simulink model "Furuta_Pendulum_Model_Revolinsky_V4"  (R2018b)
settings: Solver=ode1  StartTime=0.0  StopTime=inf  FixedStep=0.002  RelTol=1e-3  EnableMultiTasking=on
PostLoadFcn:
  | qc_set_target_type(getConfigSet(bdroot, 'QUARC Default Target Configuration'));
values from neighbouring files (symbols this model uses):
  A = zeros(4)    [Furuta_Pendulum_setup_Revolinsky.m]    (also in Furuta_Pendulum_setup_Revolinsky_edited.m; Matlab_MECA_482_SP20_Furuta_Revolinsky.m)
  a_max = T_max./(m_r.*L_r)    [Furuta_Pendulum_setup_Revolinsky.m]    (also in Furuta_Pendulum_setup_Revolinsky_edited.m; Matlab_MECA_482_SP20_Furuta_Revolinsky.m = 0)
  B = K_g * k_t * B / R_m    [Furuta_Pendulum_setup_Revolinsky.m]    (also in Furuta_Pendulum_setup_Revolinsky_edited.m; Matlab_MECA_482_SP20_Furuta_Revolinsky.m = zeros(1,4)')
  C = zeros(2,4)    [Furuta_Pendulum_setup_Revolinsky.m]    (also in Furuta_Pendulum_setup_Revolinsky_edited.m; Matlab_MECA_482_SP20_Furuta_Revolinsky.m)
  D = zeros(1,2)'    [Furuta_Pendulum_setup_Revolinsky.m]    (also in Furuta_Pendulum_setup_Revolinsky_edited.m; Matlab_MECA_482_SP20_Furuta_Revolinsky.m)
  epsilon = 12.0 * pi / 180    (= 0.209439510239)    [Furuta_Pendulum_setup_Revolinsky.m]    (also in Furuta_Pendulum_setup_Revolinsky_edited.m; Matlab_MECA_482_SP20_Furuta_Revolinsky.m)
  Er = Ep_upright_position    [Furuta_Pendulum_setup_Revolinsky.m]    (also in Furuta_Pendulum_setup_Revolinsky_edited.m; Matlab_MECA_482_SP20_Furuta_Revolinsky.m = 0)
  g = 9.81    [Furuta_Pendulum_setup_Revolinsky.m]    (also in Furuta_Pendulum_setup_Revolinsky_edited.m; Matlab_MECA_482_SP20_Furuta_Revolinsky.m)
  J_p = m_p .* L_p.^2 ./ 12    [Furuta_Pendulum_setup_Revolinsky.m]    (also in Furuta_Pendulum_setup_Revolinsky_edited.m; Matlab_MECA_482_SP20_Furuta_Revolinsky.m)
  K_g = Kgi * Kge    (= 70)    [Furuta_Pendulum_setup_Revolinsky.m]    (also in Furuta_Pendulum_setup_Revolinsky_edited.m; Matlab_MECA_482_SP20_Furuta_Revolinsky.m)
  k_m = 0.804 / 1000 * (60 / ( 2 * pi ))    (= 0.00767763445475)    [Furuta_Pendulum_setup_Revolinsky.m]    (also in Furuta_Pendulum_setup_Revolinsky_edited.m; Matlab_MECA_482_SP20_Furuta_Revolinsky.m)
  k_t = 1.088 * 0.2780139 * 0.0254    (= 0.00768296972928)    [Furuta_Pendulum_setup_Revolinsky.m]    (also in Furuta_Pendulum_setup_Revolinsky_edited.m; Matlab_MECA_482_SP20_Furuta_Revolinsky.m)
  L_p = 0.33655    [Furuta_Pendulum_setup_Revolinsky.m]    (also in Furuta_Pendulum_setup_Revolinsky_edited.m; Matlab_MECA_482_SP20_Furuta_Revolinsky.m)
  L_r = 0.2159    [Furuta_Pendulum_setup_Revolinsky.m]    (also in Furuta_Pendulum_setup_Revolinsky_edited.m; Matlab_MECA_482_SP20_Furuta_Revolinsky.m)
  m_p = 0.127    [Furuta_Pendulum_setup_Revolinsky.m]    (also in Furuta_Pendulum_setup_Revolinsky_edited.m; Matlab_MECA_482_SP20_Furuta_Revolinsky.m)
  m_r = 0.257    [Furuta_Pendulum_setup_Revolinsky.m]    (also in Furuta_Pendulum_setup_Revolinsky_edited.m; Matlab_MECA_482_SP20_Furuta_Revolinsky.m)
  n_g = 0.9    [Furuta_Pendulum_setup_Revolinsky.m]    (also in Furuta_Pendulum_setup_Revolinsky_edited.m; Matlab_MECA_482_SP20_Furuta_Revolinsky.m)
  n_m = 0.69    [Furuta_Pendulum_setup_Revolinsky.m]    (also in Furuta_Pendulum_setup_Revolinsky_edited.m; Matlab_MECA_482_SP20_Furuta_Revolinsky.m)
  R_m = 2.6    [Furuta_Pendulum_setup_Revolinsky.m]    (also in Furuta_Pendulum_setup_Revolinsky_edited.m; Matlab_MECA_482_SP20_Furuta_Revolinsky.m)
  wcf_1 = 2 * pi * 10.0    (= 62.8318530718)    [Furuta_Pendulum_setup_Revolinsky.m]    (also in Furuta_Pendulum_setup_Revolinsky_edited.m; Matlab_MECA_482_SP20_Furuta_Revolinsky.m)
  wcf_2 = 2 * pi * 10.0    (= 62.8318530718)    [Furuta_Pendulum_setup_Revolinsky.m]    (also in Furuta_Pendulum_setup_Revolinsky_edited.m; Matlab_MECA_482_SP20_Furuta_Revolinsky.m)
undefined symbols (not defined in the file or in its folder): K
libraries: simulink_extras x3, simulink x3
settings Model: ExtModeTrigDuration=10000  Creator=MLevis  LastModifiedBy=revol
settings SolverCC: PositivePriorityOrder=on
settings DataIOCC: LimitDataPoints=on  SaveFormat=Array  SignalLoggingSaveFormat=ModelDataLogs  ReturnWorkspaceOutputs=on
settings OptimizationCC: ExpressionDepthLimit=2147483647  InitFltsAndDblsToZero=on  LifeSpan=inf
settings DebuggingCC: SaveWithParameterizedLinksMsg=none  UnderspecifiedInitializationDetection=Classic  MergeDetectMultiDrivingBlocksExec=none  SolverPrmCheckMsg=warning  MultiTaskDSMMsg=warning  MultiTaskCondExecSysMsg=none  FcnCallInpInsideContextMsg=warning  StateNameClashWarn=warning  SFUnexpectedBacktrackingDiag=warning  SFNoUnconditionalDefaultTransitionDiag=warning  SFExecutionAtInitializationDiag=none
settings HardwareCC: ProdBitPerPointer=32  ProdBitPerSizeT=32  ProdBitPerPtrDiffT=32  ProdLargestAtomicFloat=None  ProdIntDivRoundTo=Undefined  ProdEndianess=Unspecified  ProdWordSize=32  ProdHWDeviceType=32-bit Generic
settings ModelReferenceCC: PropagateSignalLabelsOutOfModel=off
settings SFSimCC: SimUseLocalCustomCode=off
settings RTWCC: SystemTargetFile=quarc_win64.tlc  TemplateMakefile=quarc_default_tmf  Description=QUARC Win64 Target  RTWUseLocalCustomCode=off
settings CodeAppCC: StateflowObjectComments=on
settings STFCustomTargetCC: TargetPreCompLibLocation=C:\PROGRA~3\QUARC\lib\2018b\win64\release  GeneratePreprocessorConditionals=Disable all  CPPClassGenCompliant=on  GRTInterface=on  SystemTargetFile=quarc_win64.tlc
settings GRTTargetCC: TargetPreCompLibLocation=C:\PROGRA~3\QUARC\lib\2018b\win64\release  TargetLangStandard=C89/C90 (ANSI)  ParMdlRefBuildCompliant=off  CompOptLevelCompliant=off  ConcurrentExecutionCompliant=off  GeneratePreprocessorConditionals=Disable all  CombineOutputUpdateFcns=off  MatFileLogging=off  GRTInterface=on  UseToolchainInfoCompliant=off  ExtMode=on  ExtModeMexFile=quarc_comm
settings ConfigComp: CovMetricSettings=dw  CovHtmlReporting=on  CovSaveCumulativeToWorkspaceVar=on  CovSaveSingleToWorkspaceVar=on  CovExternalEMLEnable=off

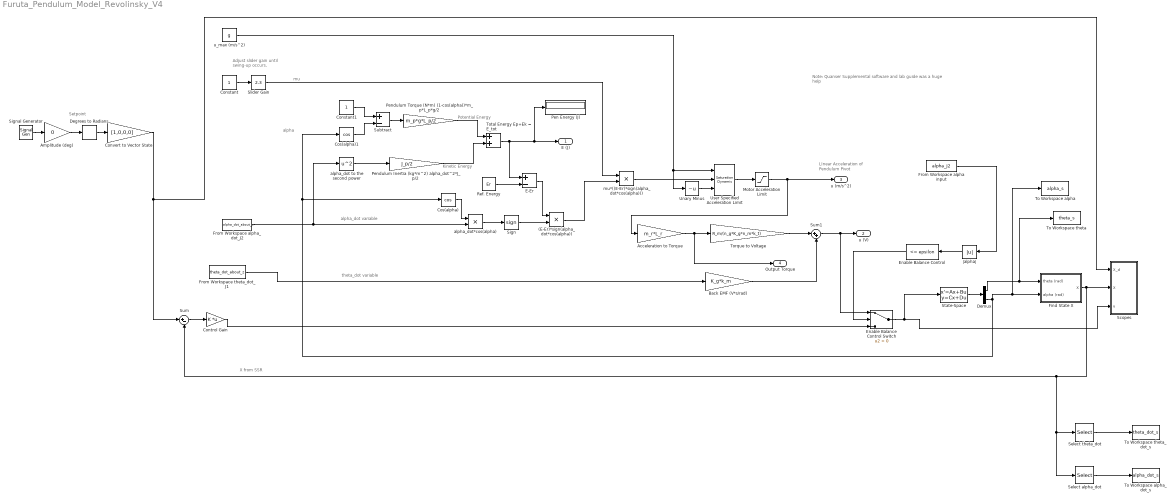
== system Furuta_Pendulum_Model_Revolinsky_V4 ==
  note: Setpoint
  note: Adjust slider gain
      | until swing-up occurs.
  note: theta_dot variable
  note: LInear Acceleration of
      | Pendulum Pivot
  note: Potential Energy
  note: Kinetic Energy
  note: alpha_dot variable
  note: X from SSR
  note: alpha
  note: mu
  note: Note: Quanser Supplemental software and lab guide was a huge help
  (E-Er)*sign(alpha_dot*cos(alpha)) : Product
  Acceleration to Torque : Gain  Gain=m_r*L_r
  Amplitude (deg) : Gain  Gain=0  SaturateOnIntegerOverflow=on  OutDataTypeStr=Inherit: Same as input  ParamDataTypeStr=Inherit: Same as input
  Back EMF (V*s/rad) : Gain  Gain=K_g*k_m
  Constant : Constant
  Constant1 : Constant
  Control Gain : Gain  Gain=K  Multiplication=Matrix(K*u)
  Convert to Vector State : Gain  Gain=[1,0,0,0]
  Cos(alpha) : Trigonometry  Operator=cos
  Cos(alpha)1 : Trigonometry  Operator=cos
  Degrees to Radians : simulink_extras/Transformations/Degrees to Radians
  Demux : Demux  Outputs=2
  E-Er : Sum  Inputs=+-
  Enable Balance Control : simulink/Logic and Bit Operations/Compare To Constant  relop=<=  const=epsilon  OutDataTypeStr=uint8  ZeroCross=off
  Enable Balance Control Switch : Switch  Criteria=u2 > Threshold
  Find State X : Subsystem
  From Workspace alpha input : FromWorkspace  VariableName=alpha_J2
  From Workspace alpha_dot_J2 : FromWorkspace  VariableName=alpha_dot_about_x
  From Workspace theta_dot_J1 : FromWorkspace  VariableName=theta_dot_about_z
  Motor Acceleration Limit : Saturate  UpperLimit=a_max  LowerLimit=-a_max
  Pen Energy (J) : Display
      settings: Decimation=100
  Pendulum Inertia (kg*m^2) alpha_dot^2*J_p/2 : Gain  Gain=J_p/2
  Pendulum Torque (N*m) (1-cos(alpha))*m_p*L_p*g/2 : Gain  Gain=m_p*g*L_p/2
  Ref. Energy : Constant  Value=Er
  Scopes : Subsystem
  Select alpha_dot : Selector  InputPortWidth=4  IndexOptions=Index vector (dialog)  Indices=[4]  OutputSizes=1
  Select theta_dot : Selector  InputPortWidth=4  IndexOptions=Index vector (dialog)  Indices=[3]  OutputSizes=1
  Sign : Signum
  Signal Generator : SignalGenerator  WaveForm=square  Frequency=0.1
  Slider Gain : simulink/Math Operations/Slider Gain  gain=2.3  low=0  high=10
  State-Space : StateSpace  A=A  B=B  C=C  D=D  InitialCondition=0
  Subtract : Sum  Inputs=+-
  Sum : Sum  Inputs=|+-
  Sum1 : Sum  Inputs=|++
  To Workspace alpha : ToWorkspace  VariableName=alpha_s  SaveFormat=Structure  SampleTime=-1
  To Workspace alpha_dot_s : ToWorkspace  VariableName=alpha_dot_s  SaveFormat=Structure  SampleTime=-1
  To Workspace theta : ToWorkspace  VariableName=theta_s  SaveFormat=Structure  SampleTime=-1
  To Workspace theta_dot_s : ToWorkspace  VariableName=theta_dot_s  SaveFormat=Structure  SampleTime=-1
  Torque to Voltage : Gain  Gain=R_m/(n_g*K_g*n_m*k_t)
  Total Energy Ep+Ek = E_tot : Sum
  Unary Minus : UnaryMinus
  User Specified Acceleration Limit : simulink/Discontinuities/Saturation Dynamic  OutMin=[]  OutMax=[]  OutDataTypeStr=Inherit: Same as second input  OutDataType=fixdt(1, 16)  OutScaling=2^-10  DoSatur=off
  alpha_dot to the second power : Math  Operator=square  SaturateOnIntegerOverflow=on
  alpha_dot*cos(alpha) : Product
  mu*((E-Er)*sign(alpha_dot*cos(alpha))) : Product
  u_max (m/s^2) : Constant  Value=g
  |alpha| : Abs
  E (J) : Outport
  u (V) : Outport  Port=2
  u (m/s^2) : Outport  Port=3
  Output Torque : Outport  Port=4
  wires:
  Amplitude (deg)/1 -> Degrees to Radians/1
  Signal Generator/1 -> Amplitude (deg)/1
  Degrees to Radians/1 -> Convert to Vector State/1
  Convert to Vector State/1 -> Sum/1, Scopes/1(X_d)
  Demux/1 -> To Workspace theta/1, Find State X/1(theta (rad))
  Sum/1 -> Control Gain/1
  |alpha|/1 -> Enable Balance Control/1
  Constant/1 -> Slider Gain/1
  Enable Balance Control/1 -> Enable Balance Control Switch/2
  Enable Balance Control Switch/1 -> State-Space/1, Scopes/3(u)
  Control Gain/1 -> Enable Balance Control Switch/3
  u_max (m/s^2)/1 -> User Specified Acceleration Limit/1, Unary Minus/1
  Demux/2 -> Cos(alpha)1/1, Cos(alpha)/1, Find State X/2(alpha (rad)), To Workspace alpha/1
  From Workspace alpha_dot_J2/1 -> alpha_dot to the second power/1, alpha_dot*cos(alpha)/2
  Slider Gain/1 -> mu*((E-Er)*sign(alpha_dot*cos(alpha)))/1
  From Workspace theta_dot_J1/1 -> Back EMF (V*s/rad)/1
  Back EMF (V*s/rad)/1 -> Sum1/2
  Ref. Energy/1 -> E-Er/2
  (E-Er)*sign(alpha_dot*cos(alpha))/1 -> mu*((E-Er)*sign(alpha_dot*cos(alpha)))/2
  mu*((E-Er)*sign(alpha_dot*cos(alpha)))/1 -> User Specified Acceleration Limit/2
  Find State X/1(X) -> Select alpha_dot/1, Select theta_dot/1, Sum/2, Scopes/2(X)
  alpha_dot*cos(alpha)/1 -> Sign/1
  alpha_dot to the second power/1 -> Pendulum Inertia (kg*m^2) alpha_dot^2*J_p/2/1
  E-Er/1 -> (E-Er)*sign(alpha_dot*cos(alpha))/1
  Torque to Voltage/1 -> Sum1/1
  Total Energy Ep+Ek = E_tot/1 -> E-Er/1, E (J)/1, Pen Energy (J)/1
  Cos(alpha)1/1 -> Subtract/2
  Acceleration to Torque/1 -> Output Torque/1, Torque to Voltage/1
  Sign/1 -> (E-Er)*sign(alpha_dot*cos(alpha))/2
  Cos(alpha)/1 -> alpha_dot*cos(alpha)/1
  Unary Minus/1 -> User Specified Acceleration Limit/3
  Pendulum Inertia (kg*m^2) alpha_dot^2*J_p/2/1 -> Total Energy Ep+Ek = E_tot/2
  Subtract/1 -> Pendulum Torque (N*m) (1-cos(alpha))*m_p*L_p*g/2/1
  Motor Acceleration Limit/1 -> Acceleration to Torque/1, u (m/s^2)/1
  User Specified Acceleration Limit/1 -> Motor Acceleration Limit/1
  Constant1/1 -> Subtract/1
  Pendulum Torque (N*m) (1-cos(alpha))*m_p*L_p*g/2/1 -> Total Energy Ep+Ek = E_tot/1
  Sum1/1 -> Enable Balance Control Switch/1, u (V)/1
  State-Space/1 -> Demux/1
  From Workspace alpha input/1 -> |alpha|/1
  Select theta_dot/1 -> To Workspace theta_dot_s/1
  Select alpha_dot/1 -> To Workspace alpha_dot_s/1

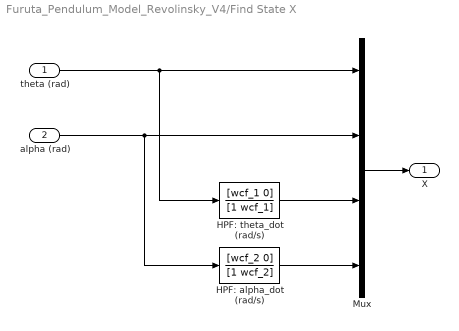
== system Furuta_Pendulum_Model_Revolinsky_V4/Find State X ==
  theta (rad) : Inport
  alpha (rad) : Inport  Port=2
  HPF: alpha_dot (rad/s) : TransferFcn  Numerator=[wcf_2 0]  Denominator=[1 wcf_2]
  HPF: theta_dot (rad/s) : TransferFcn  Numerator=[wcf_1 0]  Denominator=[1 wcf_1]
  Mux : Mux
  X : Outport
  wires:
  alpha (rad)/1 -> Mux/2, HPF: alpha_dot (rad/s)/1
  Mux/1 -> X/1
  theta (rad)/1 -> Mux/1, HPF: theta_dot (rad/s)/1
  HPF: theta_dot (rad/s)/1 -> Mux/3
  HPF: alpha_dot (rad/s)/1 -> Mux/4

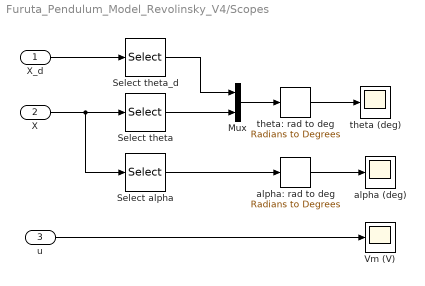
== system Furuta_Pendulum_Model_Revolinsky_V4/Scopes ==
  X_d : Inport
  X : Inport  Port=2
  u : Inport  Port=3
  Mux : Mux  Inputs=2
  Select alpha : Selector  InputPortWidth=4  IndexOptions=Index vector (dialog)  Indices=2  OutputSizes=[(-2)]
  Select theta : Selector  InputPortWidth=4  IndexOptions=Index vector (dialog)  Indices=1  OutputSizes=[(-2)]
  Select theta_d : Selector  InputPortWidth=4  IndexOptions=Index vector (dialog)  Indices=1  OutputSizes=[(-2)]
  Vm (V) : Scope
  alpha (deg) : Scope
  alpha: rad to deg : simulink_extras/Transformations/Radians to Degrees
  theta (deg) : Scope
  theta: rad to deg : simulink_extras/Transformations/Radians to Degrees
  wires:
  u/1 -> Vm (V)/1
  X_d/1 -> Select theta_d/1
  Mux/1 -> theta: rad to deg/1
  Select alpha/1 -> alpha: rad to deg/1
  alpha: rad to deg/1 -> alpha (deg)/1
  X/1 -> Select alpha/1, Select theta/1
  Select theta_d/1 -> Mux/1
  theta: rad to deg/1 -> theta (deg)/1
  Select theta/1 -> Mux/2
